simulink model "Simulador_PID_Motor"  (R2024b)
settings: Solver=VariableStepAuto  StartTime=0.0  StopTime=5  RelTol=1e-3
undefined symbols (not defined in the file): Kp1, Kp2, T, Ti
settings Model: Creator=gusta  LastModifiedBy=syaba

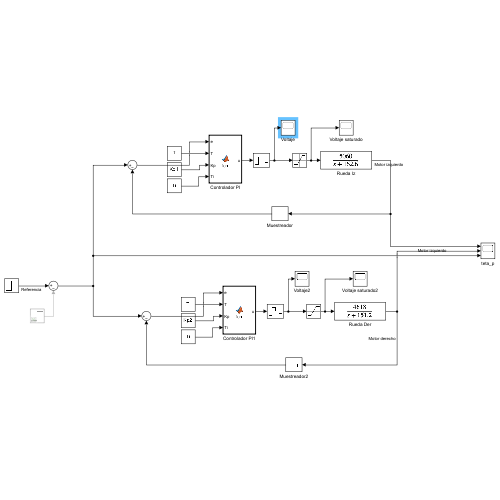
[thumbnail: Simulink's stored preview of the top-level diagram]
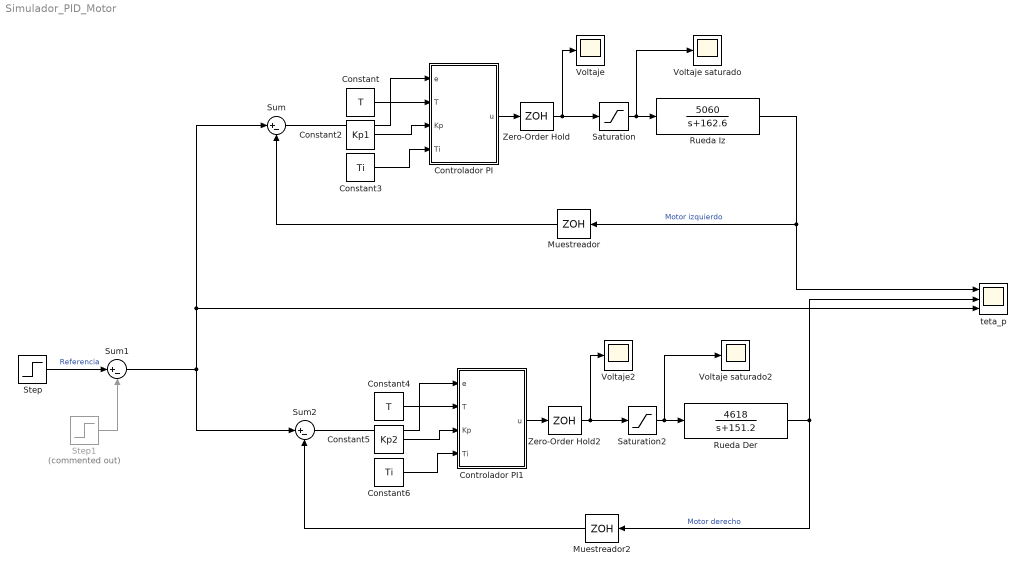
== system Simulador_PID_Motor ==
  Constant : Constant  Value=T
  Constant2 : Constant  Value=Kp1
  Constant3 : Constant  Value=Ti
  Constant4 : Constant  Value=T
  Constant5 : Constant  Value=Kp2
  Constant6 : Constant  Value=Ti
  Controlador PI : MATLAB Function  TreatAsAtomicUnit=on  SystemSampleTime=T
  Controlador PI1 : MATLAB Function  TreatAsAtomicUnit=on  SystemSampleTime=T
  Muestreador : ZeroOrderHold  SampleTime=T
  Muestreador2 : ZeroOrderHold  SampleTime=T
  Rueda Der : TransferFcn  Numerator=[4618]  Denominator=[1 151.2]
  Rueda Iz : TransferFcn  Numerator=[5060]  Denominator=[1 162.6]
  Saturation : Saturate  UpperLimit=9  LowerLimit=-9
  Saturation2 : Saturate  UpperLimit=9  LowerLimit=-9
  Step : Step  Time=0  After=275  SampleTime=0
  Step1 : Step  Commented=on  Time=5  After=275  SampleTime=0
  Sum : Sum  Inputs=|+-
  Sum1 : Sum  Inputs=|+-
  Sum2 : Sum  Inputs=|+-
  Voltaje : Scope
  Voltaje saturado : Scope
  Voltaje saturado2 : Scope
  Voltaje2 : Scope
  Zero-Order Hold : ZeroOrderHold  SampleTime=T
  Zero-Order Hold2 : ZeroOrderHold  SampleTime=T
  teta_p : Scope  NumInputPorts=3
  wires:
  Saturation/1 -> Voltaje saturado/1, Rueda Iz/1
  Constant/1 -> Controlador PI/2(T)
  Rueda Iz/1 -> Muestreador/1, teta_p/1  "Motor izquierdo"
  Sum/1 -> Controlador PI/1(e)
  Muestreador/1 -> Sum/2
  Zero-Order Hold/1 -> Saturation/1, Voltaje/1
  Controlador PI/1(u) -> Zero-Order Hold/1
  Constant2/1 -> Controlador PI/3(Kp)
  Constant3/1 -> Controlador PI/4(Ti)
  Constant5/1 -> Controlador PI1/3(Kp)
  Constant6/1 -> Controlador PI1/4(Ti)
  Sum2/1 -> Controlador PI1/1(e)
  Constant4/1 -> Controlador PI1/2(T)
  Rueda Der/1 -> Muestreador2/1, teta_p/2  "Motor derecho"
  Saturation2/1 -> Rueda Der/1, Voltaje saturado2/1
  Muestreador2/1 -> Sum2/2
  Zero-Order Hold2/1 -> Saturation2/1, Voltaje2/1
  Controlador PI1/1(u) -> Zero-Order Hold2/1
  Step/1 -> Sum1/1  "Referencia"
  Step1/1 -> Sum1/2
  Sum1/1 -> teta_p/3, Sum/1, Sum2/1

== matlab function Simulador_PID_Motor/Controlador PI ==
  data: e input; u output; T input; Kp input; Ti input
function u = fcn(e,T, Kp, Ti)

persistent I_ant;

if isempty(I_ant),
    I_ant=0;
end;

I = I_ant + e*T;

u = Kp*(e + (1/Ti)*I);

I_ant = I;

== matlab function Simulador_PID_Motor/Controlador PI1 ==
  data: e input; u output; T input; Kp input; Ti input
function u = fcn(e,T, Kp, Ti)

persistent I_ant;

if isempty(I_ant),
    I_ant=0;
end;

I = I_ant + e*T;

u = Kp*(e + (1/Ti)*I);

I_ant = I;
